simulink model "add_sub_mul"  (R2016a)
settings: Solver=VariableStepAuto  StartTime=0.0  StopTime=10.0  RelTol=1e-3
libraries: visionsources x1
settings Model: Creator=Auroshis  LastModifiedBy=Auroshis

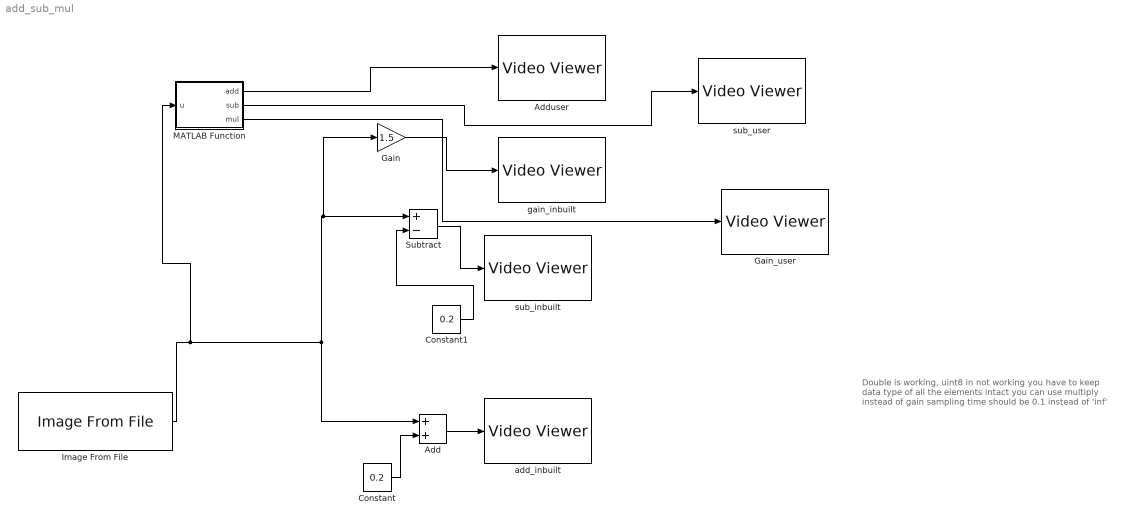
== system add_sub_mul ==
  note: Double is working, uint8 in not working
      | you have to keep data type of all the elements intact
      | you can use multiply instead of gain
      | sampling time should be 0.1 instead of 'inf'
  Add : Sum
  Adduser : VideoViewer  FigPos=[293 442.8 409.6 300]
  Constant : Constant  Value=0.2  OutDataTypeStr=uint8  SampleTime=0.1
  Constant1 : Constant  Value=0.2  OutDataTypeStr=uint8  SampleTime=0.1
  Gain : Gain  Gain=1.5  OutDataTypeStr=double
  Gain_user : VideoViewer  FigPos=[243.4 430.8 409.6 300]
  Image From File : visionsources/Image From File  Tag=vipblks_nd  FileName=cameraman.tif  imagePorts=One multidimensional signal  Ts=0.1  ImageDataType=double  Signed=on  WordLength=16  sdImageDataType=uint(8)  FractionLengthMode=User-defined  FractionLength=15  OutPortLabels=R|G|B
  MATLAB Function : MATLAB Function  TreatAsAtomicUnit=on
  Subtract : Sum  Inputs=+-
  add_inbuilt : VideoViewer  Tag=addition  FigPos=[700.2 442 409.6 300]
  gain_inbuilt : VideoViewer  FigPos=[656.2 429.2 409.6 300]
  sub_inbuilt : VideoViewer  FigPos=[655.4 838.8 409.6 300]
  sub_user : VideoViewer  FigPos=[243.4 838 409.6 300]
  wires:
  Constant/1 -> Add/2
  Constant1/1 -> Subtract/2
  Add/1 -> add_inbuilt/1
  Subtract/1 -> sub_inbuilt/1
  Gain/1 -> gain_inbuilt/1
  Image From File/1 -> MATLAB Function/1(u), Add/1, Gain/1, Subtract/1
  MATLAB Function/1(add) -> Adduser/1
  MATLAB Function/2(sub) -> sub_user/1
  MATLAB Function/3(mul) -> Gain_user/1

== matlab function add_sub_mul/MATLAB Function ==
  data: u input; add output; sub output; mul output
function [add, sub, mul]= fcn(u)
add = u + 0.2;
sub = u - 0.2;
mul = u * 1.5;
